simulink model "xy_control"  (R2018a)
settings: Solver=VariableStepAuto  StartTime=0.0  StopTime=50  RelTol=1e-3
undefined symbols (not defined in the file): drone, input_thrust_limit, input_torque_x_limit, input_torque_y_limit, input_torque_z_limit, psit, regulated_target_angular, regulated_target_velocity, regulator_gain_of_attitude, simulation_sampling_ts, target_angular_limit, target_velocity_limit, target_velocity_z_limit, vd, vi, vp, xp, xt, yp, yt, zt
libraries: simulink x6
settings Model: Creator=ros  LastModifiedBy=ros

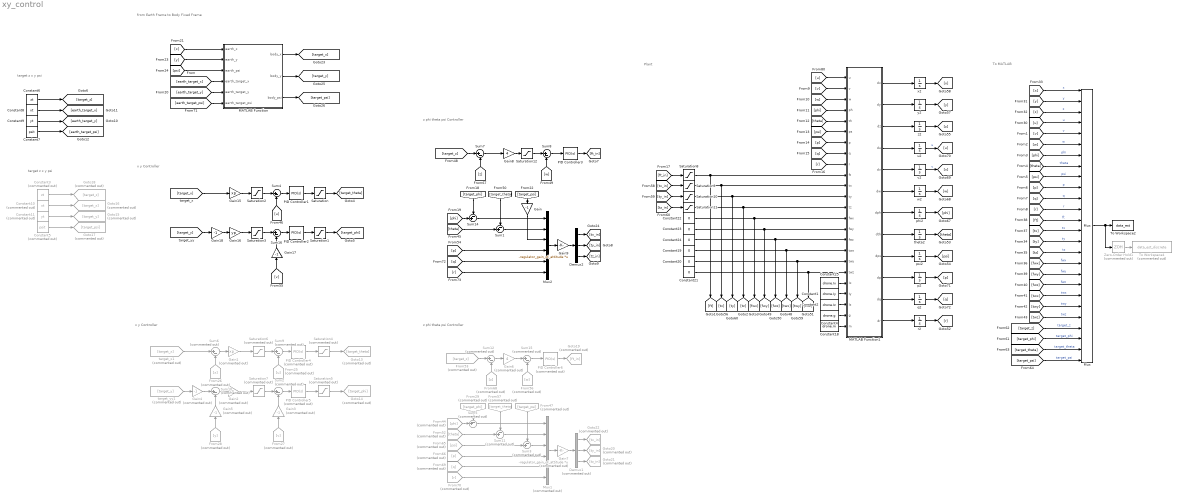
== system xy_control ==
  note: Plant
  note: To MATLAB
  note: x y Controller
  note: from Earth Frame to Body Fixed Frame
  note: target z x y psi
  note: x y Controller
  note: target z x y psi
  note: z phi theta psi Controller
  note: z phi theta psi Controller
  Constant1 : Constant  Value=drone.Iy
  Constant10 : Constant  Commented=on  Value=xt
  Constant11 : Constant  Commented=on  Value=yt
  Constant18 : Constant  Value=drone.m
  Constant{19..24} (6 alike) : Constant  Value=0
  Constant2 : Constant  Value=drone.Iz
  Constant25 : Constant  Value=drone.Ix
  Constant3 : Constant  Commented=on  Value=zt
  Constant4 : Constant  Value=drone.g
  Constant5 : Constant  Commented=on  Value=psit
  Constant6 : Constant  Value=zt
  Constant7 : Constant  Value=psit
  Constant8 : Constant  Value=xt
  Constant9 : Constant  Value=yt
  Demux1 : Demux  Commented=on  Outputs=3
  Demux2 : Demux  Outputs=3
  From25 : From  Commented=on  GotoTag=u
  From26 : From  Commented=on  GotoTag=x
  From27 : From  Commented=on  GotoTag=v
  From28 : From  Commented=on  GotoTag=y
  From29 : From  Commented=on  GotoTag=target_phi
  From44 : From  Commented=on  GotoTag=phi
  From47 : From  Commented=on  GotoTag=target_psi
  From52 : From  Commented=on  GotoTag=theta
  From53 : From  Commented=on  GotoTag=target_z
  From56 : From  Commented=on  GotoTag=w
  From57 : From  Commented=on  GotoTag=target_theta
  From65 : From  Commented=on  GotoTag=psi
  From66 : From  Commented=on  GotoTag=p
  From68 : From  Commented=on  GotoTag=z
  From69 : From  Commented=on  GotoTag=q
  From70 : From  Commented=on  GotoTag=r
  Gain : Gain  Gain=-1
  Gain1 : Gain  Commented=on  Gain=xp
  Gain15 : Gain  Gain=xp
  Gain16 : Gain  Gain=yp
  Gain17 : Gain  Gain=-1
  Gain18 : Gain  Gain=-1
  Gain2 : Gain  Commented=on  Gain=yp
  Gain3 : Gain  Commented=on  Gain=-1
  Gain4 : Gain  Commented=on  Gain=-1
  Gain5 : Gain  Commented=on  Gain=-1
  Gain6 : Gain  Commented=on  Gain=4
  Gain7 : Gain  Commented=on  Gain=-regulator_gain_of_attitude  Multiplication=Matrix(K*u)
  Gain8 : Gain  Gain=4
  Gain9 : Gain  Gain=-regulator_gain_of_attitude  Multiplication=Matrix(K*u)
  Goto13 : Goto  Commented=on  GotoTag=target_theta
  Goto14 : Goto  Commented=on  GotoTag=target_phi
  Goto15 : Goto  Commented=on  GotoTag=target_y
  Goto16 : Goto  Commented=on  GotoTag=target_x
  Goto17 : Goto  Commented=on  GotoTag=target_psi
  Goto18 : Goto  Commented=on  GotoTag=target_z
  Goto19 : Goto  Commented=on  GotoTag=ft_in
  Goto20 : Goto  Commented=on  GotoTag=ty_in
  Goto21 : Goto  Commented=on  GotoTag=tz_in
  Goto22 : Goto  Commented=on  GotoTag=tx_in
  MATLAB Function : MATLAB Function  TreatAsAtomicUnit=on
  MATLAB Function1 : MATLAB Function  TreatAsAtomicUnit=on
  Mux : Mux  Inputs=26
      settings: DisplayOption=signals
  Mux1 : Mux  Commented=on  Inputs=6
  Mux2 : Mux  Inputs=6
  PID Controller1 : simulink/Continuous/PID Controller  Controller=PID  TimeDomain=Continuous-time  SampleTime=-1  IntegratorMethod=Forward Euler  FilterMethod=Forward Euler  Form=Parallel  UseFilter=on  ControllerParametersSource=internal  P=vp  I=vi  D=vd  N=100  InitialConditionSource=internal  InitialConditionForIntegrator=0  InitialConditionForFilter=0  ExternalReset=none  LimitOutput=off  UpperSaturationLimit=inf  LowerSaturationLimit=-inf  LinearizeAsGain=on  AntiWindupMode=none  Kb=1  TrackingMode=off  Kt=1  PParamMin=[]  PParamMax=[]  IParamMin=[]  IParamMax=[]  DParamMin=[]  DParamMax=[]  NParamMin=[]  NParamMax=[]  KbParamMin=[]  KbParamMax=[]  KtParamMin=[]  KtParamMax=[]  POutMin=[]  POutMax=[]  IOutMin=[]  IOutMax=[]  DOutMin=[]  DOutMax=[]  NOutMin=[]  NOutMax=[]  KbOutMin=[]  KbOutMax=[]  KtOutMin=[]  KtOutMax=[]  IntegratorOutMin=[]  IntegratorOutMax=[]  FilterOutMin=[]  FilterOutMax=[]  SumOutMin=[]  SumOutMax=[]  SumI1OutMin=[]  SumI1OutMax=[]  SumI2OutMin=[]  SumI2OutMax=[]  SumI3OutMin=[]  SumI3OutMax=[]  SumDOutMin=[]  SumDOutMax=[]  SaturationOutMin=[]  SaturationOutMax=[]  IntegratorContinuousStateAttributes=''  IntegratorStateMustResolveToSignalObject=off  IntegratorRTWStateStorageClass=Auto  FilterContinuousStateAttributes=''  FilterStateMustResolveToSignalObject=off  FilterRTWStateStorageClass=Auto  DifferentiatorICPrevScaledInput=0  DifferentiatorOutMin=[]  DifferentiatorOutMax=[]  FilterDiffOutCoefMin=[]  FilterDiffOutCoefMax=[]  SumDenOutMin=[]  SumDenOutMax=[]  SumNumOutMin=[]  SumNumOutMax=[]  ReciprocalOutMin=[]  ReciprocalOutMax=[]  DivideOutMin=[]  DivideOutMax=[]  TunerSelectOption=Transfer Function Based (PID Tuner App)
  PID Controller2 : simulink/Continuous/PID Controller  Controller=PID  TimeDomain=Continuous-time  SampleTime=-1  IntegratorMethod=Forward Euler  FilterMethod=Forward Euler  Form=Parallel  UseFilter=on  ControllerParametersSource=internal  P=vp  I=vi  D=vd  N=113.724914636651  InitialConditionSource=internal  InitialConditionForIntegrator=0  InitialConditionForFilter=0  ExternalReset=none  LimitOutput=off  UpperSaturationLimit=inf  LowerSaturationLimit=-inf  LinearizeAsGain=on  AntiWindupMode=none  Kb=1  TrackingMode=off  Kt=1  PParamMin=[]  PParamMax=[]  IParamMin=[]  IParamMax=[]  DParamMin=[]  DParamMax=[]  NParamMin=[]  NParamMax=[]  KbParamMin=[]  KbParamMax=[]  KtParamMin=[]  KtParamMax=[]  POutMin=[]  POutMax=[]  IOutMin=[]  IOutMax=[]  DOutMin=[]  DOutMax=[]  NOutMin=[]  NOutMax=[]  KbOutMin=[]  KbOutMax=[]  KtOutMin=[]  KtOutMax=[]  IntegratorOutMin=[]  IntegratorOutMax=[]  FilterOutMin=[]  FilterOutMax=[]  SumOutMin=[]  SumOutMax=[]  SumI1OutMin=[]  SumI1OutMax=[]  SumI2OutMin=[]  SumI2OutMax=[]  SumI3OutMin=[]  SumI3OutMax=[]  SumDOutMin=[]  SumDOutMax=[]  SaturationOutMin=[]  SaturationOutMax=[]  IntegratorContinuousStateAttributes=''  IntegratorStateMustResolveToSignalObject=off  IntegratorRTWStateStorageClass=Auto  FilterContinuousStateAttributes=''  FilterStateMustResolveToSignalObject=off  FilterRTWStateStorageClass=Auto  DifferentiatorICPrevScaledInput=0  DifferentiatorOutMin=[]  DifferentiatorOutMax=[]  FilterDiffOutCoefMin=[]  FilterDiffOutCoefMax=[]  SumDenOutMin=[]  SumDenOutMax=[]  SumNumOutMin=[]  SumNumOutMax=[]  ReciprocalOutMin=[]  ReciprocalOutMax=[]  DivideOutMin=[]  DivideOutMax=[]  TunerSelectOption=Transfer Function Based (PID Tuner App)
  PID Controller3 : simulink/Continuous/PID Controller  Controller=PID  TimeDomain=Continuous-time  SampleTime=-1  IntegratorMethod=Forward Euler  FilterMethod=Forward Euler  Form=Parallel  UseFilter=on  ControllerParametersSource=internal  P=7  I=6  D=0.4  N=100  InitialConditionSource=internal  InitialConditionForIntegrator=0  InitialConditionForFilter=0  ExternalReset=none  LimitOutput=off  UpperSaturationLimit=inf  LowerSaturationLimit=-inf  LinearizeAsGain=on  AntiWindupMode=none  Kb=1  TrackingMode=off  Kt=1  PParamMin=[]  PParamMax=[]  IParamMin=[]  IParamMax=[]  DParamMin=[]  DParamMax=[]  NParamMin=[]  NParamMax=[]  KbParamMin=[]  KbParamMax=[]  KtParamMin=[]  KtParamMax=[]  POutMin=[]  POutMax=[]  IOutMin=[]  IOutMax=[]  DOutMin=[]  DOutMax=[]  NOutMin=[]  NOutMax=[]  KbOutMin=[]  KbOutMax=[]  KtOutMin=[]  KtOutMax=[]  IntegratorOutMin=[]  IntegratorOutMax=[]  FilterOutMin=[]  FilterOutMax=[]  SumOutMin=[]  SumOutMax=[]  SumI1OutMin=[]  SumI1OutMax=[]  SumI2OutMin=[]  SumI2OutMax=[]  SumI3OutMin=[]  SumI3OutMax=[]  SumDOutMin=[]  SumDOutMax=[]  SaturationOutMin=[]  SaturationOutMax=[]  IntegratorContinuousStateAttributes=''  IntegratorStateMustResolveToSignalObject=off  IntegratorRTWStateStorageClass=Auto  FilterContinuousStateAttributes=''  FilterStateMustResolveToSignalObject=off  FilterRTWStateStorageClass=Auto  DifferentiatorICPrevScaledInput=0  DifferentiatorOutMin=[]  DifferentiatorOutMax=[]  FilterDiffOutCoefMin=[]  FilterDiffOutCoefMax=[]  SumDenOutMin=[]  SumDenOutMax=[]  SumNumOutMin=[]  SumNumOutMax=[]  ReciprocalOutMin=[]  ReciprocalOutMax=[]  DivideOutMin=[]  DivideOutMax=[]  TunerSelectOption=Transfer Function Based (PID Tuner App)
  PID Controller4 : simulink/Continuous/PID Controller  Commented=on  Controller=PID  TimeDomain=Continuous-time  SampleTime=-1  IntegratorMethod=Forward Euler  FilterMethod=Forward Euler  Form=Parallel  UseFilter=on  ControllerParametersSource=internal  P=vp  I=vi  D=vd  N=100  InitialConditionSource=internal  InitialConditionForIntegrator=0  InitialConditionForFilter=0  ExternalReset=none  LimitOutput=off  UpperSaturationLimit=inf  LowerSaturationLimit=-inf  LinearizeAsGain=on  AntiWindupMode=none  Kb=1  TrackingMode=off  Kt=1  PParamMin=[]  PParamMax=[]  IParamMin=[]  IParamMax=[]  DParamMin=[]  DParamMax=[]  NParamMin=[]  NParamMax=[]  KbParamMin=[]  KbParamMax=[]  KtParamMin=[]  KtParamMax=[]  POutMin=[]  POutMax=[]  IOutMin=[]  IOutMax=[]  DOutMin=[]  DOutMax=[]  NOutMin=[]  NOutMax=[]  KbOutMin=[]  KbOutMax=[]  KtOutMin=[]  KtOutMax=[]  IntegratorOutMin=[]  IntegratorOutMax=[]  FilterOutMin=[]  FilterOutMax=[]  SumOutMin=[]  SumOutMax=[]  SumI1OutMin=[]  SumI1OutMax=[]  SumI2OutMin=[]  SumI2OutMax=[]  SumI3OutMin=[]  SumI3OutMax=[]  SumDOutMin=[]  SumDOutMax=[]  SaturationOutMin=[]  SaturationOutMax=[]  IntegratorContinuousStateAttributes=''  IntegratorStateMustResolveToSignalObject=off  IntegratorRTWStateStorageClass=Auto  FilterContinuousStateAttributes=''  FilterStateMustResolveToSignalObject=off  FilterRTWStateStorageClass=Auto  DifferentiatorICPrevScaledInput=0  DifferentiatorOutMin=[]  DifferentiatorOutMax=[]  FilterDiffOutCoefMin=[]  FilterDiffOutCoefMax=[]  SumDenOutMin=[]  SumDenOutMax=[]  SumNumOutMin=[]  SumNumOutMax=[]  ReciprocalOutMin=[]  ReciprocalOutMax=[]  DivideOutMin=[]  DivideOutMax=[]  TunerSelectOption=Transfer Function Based (PID Tuner App)
  PID Controller5 : simulink/Continuous/PID Controller  Commented=on  Controller=PID  TimeDomain=Continuous-time  SampleTime=-1  IntegratorMethod=Forward Euler  FilterMethod=Forward Euler  Form=Parallel  UseFilter=on  ControllerParametersSource=internal  P=vp  I=vi  D=vd  N=113.724914636651  InitialConditionSource=internal  InitialConditionForIntegrator=0  InitialConditionForFilter=0  ExternalReset=none  LimitOutput=off  UpperSaturationLimit=inf  LowerSaturationLimit=-inf  LinearizeAsGain=on  AntiWindupMode=none  Kb=1  TrackingMode=off  Kt=1  PParamMin=[]  PParamMax=[]  IParamMin=[]  IParamMax=[]  DParamMin=[]  DParamMax=[]  NParamMin=[]  NParamMax=[]  KbParamMin=[]  KbParamMax=[]  KtParamMin=[]  KtParamMax=[]  POutMin=[]  POutMax=[]  IOutMin=[]  IOutMax=[]  DOutMin=[]  DOutMax=[]  NOutMin=[]  NOutMax=[]  KbOutMin=[]  KbOutMax=[]  KtOutMin=[]  KtOutMax=[]  IntegratorOutMin=[]  IntegratorOutMax=[]  FilterOutMin=[]  FilterOutMax=[]  SumOutMin=[]  SumOutMax=[]  SumI1OutMin=[]  SumI1OutMax=[]  SumI2OutMin=[]  SumI2OutMax=[]  SumI3OutMin=[]  SumI3OutMax=[]  SumDOutMin=[]  SumDOutMax=[]  SaturationOutMin=[]  SaturationOutMax=[]  IntegratorContinuousStateAttributes=''  IntegratorStateMustResolveToSignalObject=off  IntegratorRTWStateStorageClass=Auto  FilterContinuousStateAttributes=''  FilterStateMustResolveToSignalObject=off  FilterRTWStateStorageClass=Auto  DifferentiatorICPrevScaledInput=0  DifferentiatorOutMin=[]  DifferentiatorOutMax=[]  FilterDiffOutCoefMin=[]  FilterDiffOutCoefMax=[]  SumDenOutMin=[]  SumDenOutMax=[]  SumNumOutMin=[]  SumNumOutMax=[]  ReciprocalOutMin=[]  ReciprocalOutMax=[]  DivideOutMin=[]  DivideOutMax=[]  TunerSelectOption=Transfer Function Based (PID Tuner App)
  PID Controller6 : simulink/Continuous/PID Controller  Commented=on  Controller=PID  TimeDomain=Continuous-time  SampleTime=-1  IntegratorMethod=Forward Euler  FilterMethod=Forward Euler  Form=Parallel  UseFilter=on  ControllerParametersSource=internal  P=7  I=6  D=0.7  N=100  InitialConditionSource=internal  InitialConditionForIntegrator=0  InitialConditionForFilter=0  ExternalReset=none  LimitOutput=off  UpperSaturationLimit=inf  LowerSaturationLimit=-inf  LinearizeAsGain=on  AntiWindupMode=none  Kb=1  TrackingMode=off  Kt=1  PParamMin=[]  PParamMax=[]  IParamMin=[]  IParamMax=[]  DParamMin=[]  DParamMax=[]  NParamMin=[]  NParamMax=[]  KbParamMin=[]  KbParamMax=[]  KtParamMin=[]  KtParamMax=[]  POutMin=[]  POutMax=[]  IOutMin=[]  IOutMax=[]  DOutMin=[]  DOutMax=[]  NOutMin=[]  NOutMax=[]  KbOutMin=[]  KbOutMax=[]  KtOutMin=[]  KtOutMax=[]  IntegratorOutMin=[]  IntegratorOutMax=[]  FilterOutMin=[]  FilterOutMax=[]  SumOutMin=[]  SumOutMax=[]  SumI1OutMin=[]  SumI1OutMax=[]  SumI2OutMin=[]  SumI2OutMax=[]  SumI3OutMin=[]  SumI3OutMax=[]  SumDOutMin=[]  SumDOutMax=[]  SaturationOutMin=[]  SaturationOutMax=[]  IntegratorContinuousStateAttributes=''  IntegratorStateMustResolveToSignalObject=off  IntegratorRTWStateStorageClass=Auto  FilterContinuousStateAttributes=''  FilterStateMustResolveToSignalObject=off  FilterRTWStateStorageClass=Auto  DifferentiatorICPrevScaledInput=0  DifferentiatorOutMin=[]  DifferentiatorOutMax=[]  FilterDiffOutCoefMin=[]  FilterDiffOutCoefMax=[]  SumDenOutMin=[]  SumDenOutMax=[]  SumNumOutMin=[]  SumNumOutMax=[]  ReciprocalOutMin=[]  ReciprocalOutMax=[]  DivideOutMin=[]  DivideOutMax=[]  TunerSelectOption=Transfer Function Based (PID Tuner App)
  Saturation : Saturate  UpperLimit=target_angular_limit  LowerLimit=-target_angular_limit
  Saturation1 : Saturate  UpperLimit=target_angular_limit  LowerLimit=-target_angular_limit
  Saturation10 : Saturate  UpperLimit=input_torque_y_limit  LowerLimit=-input_torque_y_limit
  Saturation11 : Saturate  UpperLimit=input_torque_z_limit  LowerLimit=-input_torque_z_limit
  Saturation12 : Saturate  UpperLimit=target_velocity_z_limit  LowerLimit=-target_velocity_z_limit
  Saturation2 : Saturate  UpperLimit=target_velocity_limit  LowerLimit=-target_velocity_limit
  Saturation3 : Saturate  UpperLimit=target_velocity_limit  LowerLimit=-target_velocity_limit
  Saturation4 : Saturate  Commented=on  UpperLimit=regulated_target_angular  LowerLimit=-regulated_target_angular
  Saturation5 : Saturate  Commented=on  UpperLimit=regulated_target_angular  LowerLimit=-regulated_target_angular
  Saturation6 : Saturate  Commented=on  UpperLimit=regulated_target_velocity  LowerLimit=-regulated_target_velocity
  Saturation7 : Saturate  Commented=on  UpperLimit=regulated_target_velocity  LowerLimit=-regulated_target_velocity
  Saturation8 : Saturate  UpperLimit=input_thrust_limit  LowerLimit=-input_thrust_limit
  Saturation9 : Saturate  UpperLimit=input_torque_x_limit  LowerLimit=-input_torque_x_limit
  Sum1 : Sum  Inputs=-+|
  Sum{2,6,9..10,12,15} (6 alike) : Sum  Commented=on  Inputs=|+-
  Sum11 : Sum  Commented=on  Inputs=-+|
  Sum14 : Sum  Inputs=-+|
  Sum{4,7..8,16} (4 alike) : Sum  Inputs=|+-
  Sum3 : Sum  Commented=on  Inputs=-+|
  Sum5 : Sum  Commented=on  Inputs=-+|
  To Workspace2 : ToWorkspace  VariableName=data_est  SaveFormat=Timeseries  SampleTime=-1
  To Workspace4 : ToWorkspace  Commented=on  VariableName=data_est_discrete  SaveFormat=Timeseries  SampleTime=-1
  Zero-Order Hold1 : ZeroOrderHold  Commented=on  SampleTime=simulation_sampling_ts
  p2 : Integrator
  phi2 : Integrator
  psi2 : Integrator  InitialCondition=0*pi/180
  q2 : Integrator
  r2 : Integrator
  target_x1 : From  Commented=on  GotoTag=target_x
  target_yy1 : From  Commented=on  GotoTag=target_y
  theta2 : Integrator
  u2 : Integrator
  v2 : Integrator
  w2 : Integrator
  x2 : Integrator
  y2 : Integrator
  z2 : Integrator
  wires:
  [x] -> Mux/1  "x"
  [v] -> Mux/5  "v"
  [z] -> Mux/3  "z"
  [w] -> Mux/6  "w"
  [p] -> Mux/10  "p"
  [phi] -> Mux/7  "phi"
  [theta] -> Mux/8  "theta"
  [r] -> Mux/12  "r"
  [y] -> Mux/2  "y"
  [psi] -> Mux/9  "psi"
  [u] -> Mux/4  "u"
  [q] -> Mux/11  "q"
  Mux/1 -> Zero-Order Hold1/1, To Workspace2/1
  [ft] -> Mux/13  "ft"
  [tx] -> Mux/14  "tx"
  [ty] -> Mux/15  "ty"
  [tz] -> Mux/16  "tz"
  [fwx] -> Mux/17  "fwx"
  [fwy] -> Mux/18  "fwy"
  [fwz] -> Mux/19  "fwz"
  [twx] -> Mux/20  "twx"
  [twy] -> Mux/21  "twy"
  [twz] -> Mux/22  "twz"
  Zero-Order Hold1/1 -> To Workspace4/1
  [target_z] -> Mux/23  "target_z"
  [target_phi] -> Mux/24  "target_phi"
  [target_theta] -> Mux/25  "target_theta"
  [target_psi] -> Mux/26  "target_psi"
  Constant20/1 -> [twy], MATLAB Function1/18(twy)
  [q] -> MATLAB Function1/8(q)
  [tz_in] -> Saturation11/1
  Constant19/1 -> [twx], MATLAB Function1/17(twx)
  Constant25/1 -> MATLAB Function1/20(Ix)
  z2/1 -> [z]
  Constant21/1 -> [twz], MATLAB Function1/19(twz)
  p2/1 -> [p]
  [theta] -> MATLAB Function1/5(th)
  r2/1 -> [r]
  [tx_in] -> Saturation9/1
  w2/1 -> [w]
  [p] -> MATLAB Function1/7(p)
  u2/1 -> [u]  "u"
  [ty_in] -> Saturation10/1
  Constant23/1 -> [fwy], MATLAB Function1/15(fwy)
  psi2/1 -> [psi]
  MATLAB Function1/1(dx) -> x2/1
  Constant1/1 -> MATLAB Function1/21(Iy)
  MATLAB Function1/5(dv) -> v2/1
  phi2/1 -> [phi]
  q2/1 -> [q]
  [psi] -> MATLAB Function1/6(ps)
  x2/1 -> [x]
  MATLAB Function1/12(dr) -> r2/1
  MATLAB Function1/8(dth) -> theta2/1
  MATLAB Function1/3(dz) -> z2/1
  MATLAB Function1/6(dw) -> w2/1
  Constant24/1 -> [fwz], MATLAB Function1/16(fwz)
  MATLAB Function1/9(dps) -> psi2/1
  y2/1 -> [y]
  [ft_in] -> Saturation8/1
  [w] -> MATLAB Function1/3(w)
  MATLAB Function1/10(dp) -> p2/1
  [phi] -> MATLAB Function1/4(ph)
  Constant4/1 -> MATLAB Function1/23(g)
  [r] -> MATLAB Function1/9(r)
  Constant18/1 -> MATLAB Function1/24(m)
  v2/1 -> [v]  "v"
  MATLAB Function1/11(dq) -> q2/1
  MATLAB Function1/4(du) -> u2/1
  theta2/1 -> [theta]
  MATLAB Function1/2(dy) -> y2/1
  [v] -> MATLAB Function1/2(v)
  MATLAB Function1/7(dph) -> phi2/1
  [u] -> MATLAB Function1/1(u)
  Constant2/1 -> MATLAB Function1/22(Iz)
  Constant22/1 -> [fwx], MATLAB Function1/14(fwx)
  [v] -> Gain17/1
  Gain16/1 -> Saturation3/1
  PID Controller1/1 -> Saturation/1
  [target_x] -> Gain15/1
  Gain17/1 -> Sum16/2
  Gain15/1 -> Saturation2/1
  PID Controller2/1 -> Saturation1/1
  Gain18/1 -> Gain16/1
  [target_y] -> Gain18/1
  [u] -> Sum4/2
  Saturation/1 -> [target_theta]
  Saturation1/1 -> [target_phi]
  Sum4/1 -> PID Controller1/1
  Sum16/1 -> PID Controller2/1
  Saturation2/1 -> Sum4/1
  Saturation3/1 -> Sum16/1
  [x] -> MATLAB Function/1(earth_x)
  [y] -> MATLAB Function/2(earth_y)
  [psi] -> MATLAB Function/3(earth_psi)
  Constant7/1 -> [earth_target_psi]
  Constant8/1 -> [earth_target_x]
  Constant9/1 -> [earth_target_y]
  Constant6/1 -> [target_z]
  Gain1/1 -> Saturation6/1
  Sum2/1 -> PID Controller5/1
  Saturation4/1 -> Goto13/1
  PID Controller4/1 -> Saturation4/1
  PID Controller5/1 -> Saturation5/1
  From28/1 -> Gain5/1
  From26/1 -> Sum6/2
  Saturation5/1 -> Goto14/1
  Sum9/1 -> PID Controller4/1
  Saturation7/1 -> Sum2/1
  Gain4/1 -> Sum10/1
  Gain2/1 -> Saturation7/1
  Saturation6/1 -> Sum9/1
  Sum10/1 -> Gain2/1
  Gain5/1 -> Sum10/2
  From27/1 -> Gain3/1
  Sum6/1 -> Gain1/1
  target_yy1/1 -> Gain4/1
  Gain3/1 -> Sum2/2
  target_x1/1 -> Sum6/1
  From25/1 -> Sum9/2
  Constant5/1 -> Goto17/1
  Constant3/1 -> Goto18/1
  Constant10/1 -> Goto16/1
  Constant11/1 -> Goto15/1
  From70/1 -> Mux1/6
  Sum12/1 -> Gain6/1
  Demux1/3 -> Goto21/1
  From52/1 -> Sum11/2
  From57/1 -> Sum11/1
  Gain7/1 -> Demux1/1
  From68/1 -> Sum12/2
  From69/1 -> Mux1/5
  Gain6/1 -> Sum15/1
  Mux1/1 -> Gain7/1
  Sum11/1 -> Mux1/2
  From47/1 -> Sum3/1
  Sum3/1 -> Mux1/3
  Demux1/1 -> Goto22/1
  From56/1 -> Sum15/2
  From53/1 -> Sum12/1
  From65/1 -> Sum3/2
  PID Controller6/1 -> Goto19/1
  Sum15/1 -> PID Controller6/1
  From66/1 -> Mux1/4
  From29/1 -> Sum5/1
  Sum5/1 -> Mux1/1
  Demux1/2 -> Goto20/1
  From44/1 -> Sum5/2
  [earth_target_x] -> MATLAB Function/4(earth_target_x)
  [earth_target_y] -> MATLAB Function/5(earth_target_y)
  [earth_target_psi] -> MATLAB Function/6(earth_target_psi)
  MATLAB Function/1(body_x) -> [target_x]
  Mux2/1 -> Gain9/1
  Gain8/1 -> Saturation12/1
  Sum14/1 -> Mux2/1
  Gain9/1 -> Demux2/1
  Sum8/1 -> PID Controller3/1
  Sum7/1 -> Gain8/1
  [target_theta] -> Sum1/1
  PID Controller3/1 -> [ft_in]
  [phi] -> Sum14/2
  [theta] -> Sum1/2
  Demux2/2 -> [ty_in]
  Demux2/3 -> [tz_in]
  [target_z] -> Sum7/1
  Sum1/1 -> Mux2/2
  Demux2/1 -> [tx_in]
  [z] -> Sum7/2
  [p] -> Mux2/4
  [q] -> Mux2/5
  [target_phi] -> Sum14/1
  [r] -> Mux2/6
  Gain/1 -> Mux2/3
  [w] -> Sum8/2
  [target_psi] -> Gain/1
  MATLAB Function/2(body_y) -> [target_y]
  MATLAB Function/3(body_psi) -> [target_psi]
  Saturation8/1 -> [ft], MATLAB Function1/10(ft)
  Saturation9/1 -> [tx], MATLAB Function1/11(tx)
  Saturation10/1 -> [ty], MATLAB Function1/12(ty)
  Saturation11/1 -> [tz], MATLAB Function1/13(tz)
  Saturation12/1 -> Sum8/1

== matlab function xy_control/MATLAB Function1 ==
  data: u input; v input; dx output; w input; ph input; th input; ps input; p input; q input; r input; ft input; tx input; ty input; tz input; fwx input; fwy input; fwz input; twx input; twy input; twz input; dy output; dz output; du output; dv output; dw output; dph output; dth output; dps output; dp output; dq output; dr output; Ix input; Iy input; Iz input; g input; m input
function [dx, dy, dz, du, dv, dw, dph, dth, dps, dp, dq, dr] = fcn(u, v, w, ph, th, ps, p, q, r, ft, tx, ty, tz, fwx, fwy, fwz, twx, twy, twz, Ix, Iy, Iz, g, m)

dx = w*(sin(ph)*sin(ps) + cos(ph)*cos(ps)*sin(th)) - v*(cos(ph)*sin(ps) - cos(ps)*sin(ph)*sin(th)) + u*(cos(ps)*cos(th));
dy = v*(cos(ph)*cos(ps) + sin(ph)*sin(ps)*sin(th)) - w*(cos(ps)*sin(ph) - cos(ph)*sin(ps)*sin(th)) + u*(cos(th)*sin(ps));
dz = w*(cos(ph)*cos(th)) - u*(sin(th)) + v*(cos(th)*sin(ph));
du = r*v - q*w + g*(sin(th)) + fwx / m;
dv = p*w - r*u - g*(sin(ph)*cos(th)) + fwy / m;
dw = q*u - p*v - g*(cos(th)*cos(ph)) + (fwz + ft) / m;
dph = p + r*(cos(ph)*tan(th)) + q*(sin(ph)*tan(th));
dth = q*(cos(th)) - r*(sin(ph));
dps = r*(cos(ph)/cos(th)) + q*(sin(ph)/cos(th));
dp = r*q*(Iy - Iz)/Ix + (tx + twx)/Ix;
dq = p*r*(Iz - Ix)/Iy + (ty + twy)/Iy;
dr = p*q*(Ix - Iy)/Iz + (tz + twz)/Iz;

== matlab function xy_control/MATLAB Function ==
  data: earth_x input; body_x output; earth_y input; earth_psi input; body_y output; earth_target_x input; earth_target_y input; earth_target_psi input; body_psi output
function [body_x, body_y, body_psi] = fcn(earth_x, earth_y, earth_psi, earth_target_x, earth_target_y, earth_target_psi)

cp = cos(earth_psi);
sp = sin(earth_psi);
earth_err_x = earth_target_x - earth_x;
earth_err_y = earth_target_y - earth_y;
body_x = earth_err_x*cp - earth_err_y*sp;
body_y = earth_err_x*sp + earth_err_y*cp;
body_psi = earth_target_psi - earth_psi;
